simulink subsystem "parktrn"  (R2020a)
settings: Solver=VariableStepAuto  StartTime=0.0  StopTime=10.0  RelTol=1e-3
libraries: simulink x1
settings Model: Creator=ZhuanZ（无密码）  LastModifiedBy=ZhuanZ（无密码）

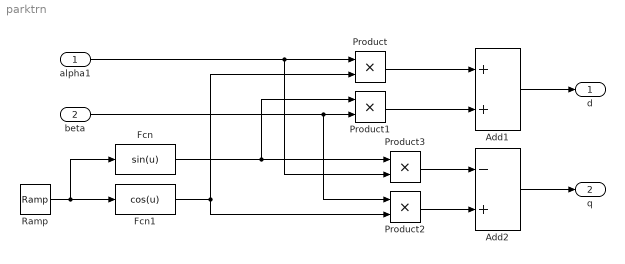
== system parktrn ==
  alpha1 : Inport
  beta : Inport  Port=2
  Add1 : Sum
  Add2 : Sum  Inputs=-+
  Fcn : Fcn  Expr=sin(u)
  Fcn1 : Fcn  Expr=cos(u)
  Product{,1..3} (4 alike) : Product  RndMeth=Zero
  Ramp : simulink/Sources/Ramp  slope=1  start=0  InitialOutput=0
  d : Outport
  q : Outport  Port=2
  wires:
  Ramp/1 -> Fcn1/1, Fcn/1
  Product/1 -> Add1/1
  Fcn1/1 -> Product2/2, Product/2
  Product3/1 -> Add2/1
  Product2/1 -> Add2/2
  Fcn/1 -> Product1/1, Product3/1
  Add2/1 -> q/1
  alpha1/1 -> Product/1, Product3/2
  beta/1 -> Product2/1, Product1/2
  Product1/1 -> Add1/2
  Add1/1 -> d/1
